simulink model "Project_FIS"  (R2018a)
settings: Solver=VariableStepAuto  StartTime=0.0  StopTime=80  RelTol=1e-3
libraries: fuzblock x1
settings Model: Creator=Wa'el WMJ  LastModifiedBy=Wa'el WMJ
settings DataIOCC: ReturnWorkspaceOutputs=on
settings DebuggingCC: UnconnectedInputMsg=none  UnconnectedOutputMsg=none  UnconnectedLineMsg=none
settings ModelReferenceCC: EnableRefExpFcnMdlSchedulingChecks=off
settings SFSimCC: SimUseLocalCustomCode=on
settings RTWCC: Description=Generic Real-Time Target  RTWUseLocalCustomCode=on

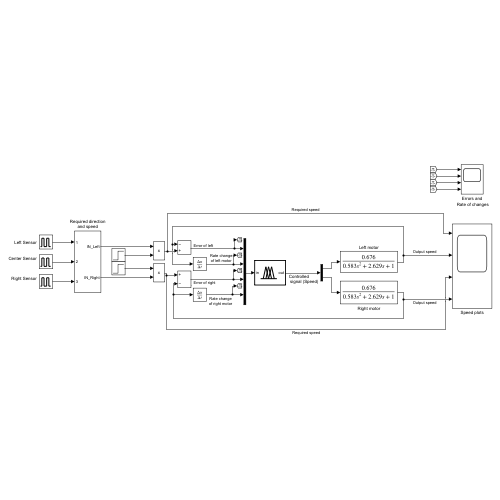
[thumbnail: Simulink's stored preview of the top-level diagram]
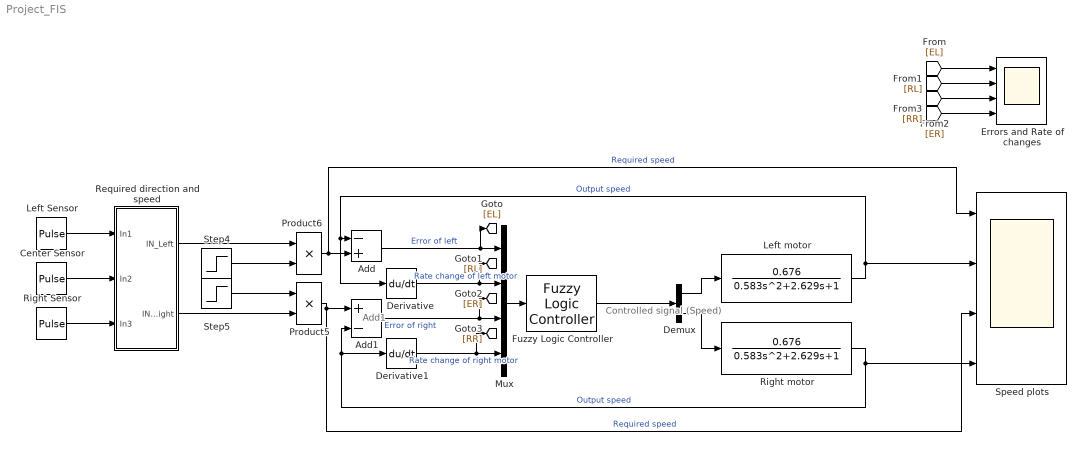
== system Project_FIS ==
  note: Controlled
      |  signal (Speed)
  note: Add1
  Add : Sum  Inputs=-+
  Add1 : Sum  Inputs=+-
  "Center Sensor " : DiscretePulseGenerator  PulseType=Time based  Period=40  PulseWidth=50  PhaseDelay=20
  Demux : Demux  Outputs=2
  Derivative : Derivative
  Derivative1 : Derivative
  Errors and Rate of changes : Scope  NumInputPorts=4
  Fuzzy Logic Controller : fuzblock/Fuzzy Logic  Controller  FIS=Speed_FIS  OutputSampleNumber=101  DataType=double  FuzzifiedInputs=off  RuleFiringStrengths=off  RuleOutputs=off  AggregatedOutputs=off  SimulateUsing=Interpreted execution  OutOfRangeInputValueMessage=warning  NoRuleFiredMessage=warning  EmptyOutputFuzzySetMessage=warning
  Left Sensor : DiscretePulseGenerator  PulseType=Time based  Period=80  PulseWidth=50  PhaseDelay=40
  Left motor : TransferFcn  Numerator=[0.676]  Denominator=[0.583 2.629 1]
  Mux : Mux
  Product5 : Product
  Product6 : Product
  Required direction and speed : Subsystem
  "Right Sensor " : DiscretePulseGenerator  PulseType=Time based  Period=20  PulseWidth=50  PhaseDelay=10
  Right motor : TransferFcn  Numerator=[0.676]  Denominator=[0.583 2.629 1]
  Speed plots : Scope  NumInputPorts=4
  Step4 : Step  Time=0  SampleTime=0
  Step5 : Step  Time=0  SampleTime=0
  wires:
  Product6/1 -> Add/2, Speed plots/1  "Required speed"
  Mux/1 -> Fuzzy Logic Controller/1
  Fuzzy Logic Controller/1 -> Demux/1
  Derivative1/1 -> [RR], Mux/4  "Rate change of right motor"
  Add1/1 -> [ER], Mux/3  "Error of right"
  Demux/2 -> Right motor/1
  Demux/1 -> Left motor/1
  Derivative/1 -> [RL], Mux/2  "Rate change of left motor"
  Left motor/1 -> Add/1, Derivative/1, Speed plots/2  "Output speed"
  Add/1 -> [EL], Mux/1  "Error of left"
  Right motor/1 -> Derivative1/1, Add1/2, Speed plots/4  "Output speed"
  Required direction and speed/1(IN_Left) -> Product6/1
  Left Sensor/1 -> Required direction and speed/1(In1)
  "Right Sensor "/1 -> Required direction and speed/3(In3)
  Required direction and speed/2(IN_Right) -> Product5/2
  Step4/1 -> Product6/2
  Step5/1 -> Product5/1
  "Center Sensor "/1 -> Required direction and speed/2(In2)
  Product5/1 -> Speed plots/3, Add1/1  "Required speed"
  [EL] -> Errors and Rate of changes/1
  [RL] -> Errors and Rate of changes/2
  [ER] -> Errors and Rate of changes/3
  [RR] -> Errors and Rate of changes/4

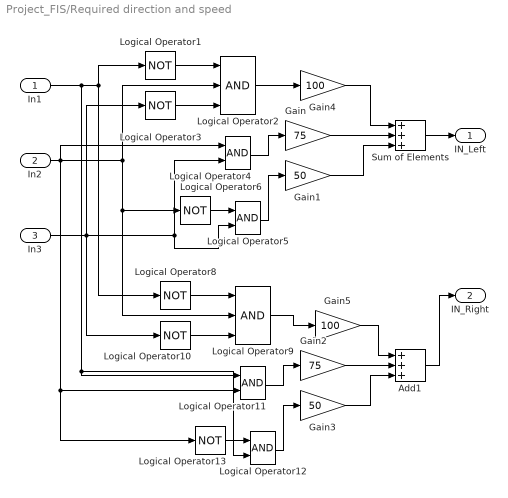
== system Project_FIS/Required direction and speed ==
  In1 : Inport
  In2 : Inport  Port=2
  In3 : Inport  Port=3
  Add1 : Sum  Inputs=+++
  Gain : Gain  Gain=75
  Gain1 : Gain  Gain=50
  Gain2 : Gain  Gain=75
  Gain3 : Gain  Gain=50
  Gain4 : Gain  Gain=100
  Gain5 : Gain  Gain=100
  Logical Operator{1,3,6,8,10,13} (6 alike) : Logic  Operator=NOT  Inputs=3  AllPortsSameDT=off  OutDataTypeStr=boolean
  Logical Operator{4..5,11..12} (4 alike) : Logic  AllPortsSameDT=off  OutDataTypeStr=boolean
  Logical Operator2 : Logic  Inputs=3  AllPortsSameDT=off  OutDataTypeStr=boolean
  Logical Operator9 : Logic  Inputs=3  AllPortsSameDT=off  OutDataTypeStr=boolean
  Sum of Elements : Sum  Inputs=+++
  IN_Left : Outport
  IN_Right : Outport  Port=2
  wires:
  Logical Operator1/1 -> Logical Operator2/1
  Logical Operator3/1 -> Logical Operator2/3
  In1/1 -> Logical Operator12/2, Logical Operator11/1, Logical Operator8/1, Logical Operator1/1
  In2/1 -> Logical Operator13/1, Logical Operator11/2, Logical Operator4/1, Logical Operator9/2, Logical Operator6/1, Logical Operator2/2
  In3/1 -> Logical Operator10/1, Logical Operator5/2, Logical Operator4/2, Logical Operator3/1
  Logical Operator6/1 -> Logical Operator5/1
  Logical Operator4/1 -> Gain/1
  Logical Operator5/1 -> Gain1/1
  Logical Operator11/1 -> Gain2/1
  Gain2/1 -> Add1/2
  Logical Operator10/1 -> Logical Operator9/3
  Logical Operator8/1 -> Logical Operator9/1
  Gain3/1 -> Add1/3
  Logical Operator12/1 -> Gain3/1
  Logical Operator13/1 -> Logical Operator12/1
  Add1/1 -> IN_Right/1
  Sum of Elements/1 -> IN_Left/1
  Gain/1 -> Sum of Elements/2
  Gain1/1 -> Sum of Elements/3
  Gain4/1 -> Sum of Elements/1
  Logical Operator2/1 -> Gain4/1
  Gain5/1 -> Add1/1
  Logical Operator9/1 -> Gain5/1
